simulink model "control_MI_dspic"  (R2018a)
settings: Solver=FixedStepAuto  StartTime=0.0  StopTime=4  FixedStep=Ts  RelTol=1e-5  EnableMultiTasking=on
PreLoadFcn:
  | inicio
InitFcn:
  | mex control_MI_dspic_main.c
values from neighbouring files (symbols this model uses):
  a = ((Llr+Lm).^2.*Rs + Lm.^2.*Rr) ./ (b.*(Llr+Lm))    [param_MI_LV.m]    (also in param_MI_VEU.m)
  A_s = 1.12    [param_veu.m]
  A_v = 1.4    [param_veu.m]
  B = 0.005752    [param_MI_LV.m]    (also in param_veu.m = 1.02)
  b = (Lls+Lm).*(Llr+Lm)-Lm.^2    [param_MI_LV.m]    (also in param_MI_VEU.m)
  B_s = (K_s/d_s)^(1/n_s)    (= 40.3936451136)    [param_veu.m]
  C = 0.68    [param_veu.m]
  C_d = 0.5    [param_veu.m]
  C_r = 0    [param_veu.m]
  C_s = 0.625    [param_veu.m]
  D_s = 1    [param_veu.m]
  eta_t = 0.9    [param_veu.m]
  g = 9.81    [param_veu.m]
  H = 0.47    [param_veu.m]
  H_a = H    (= 0.47)    [param_veu.m]
  J_m = 0.02    [param_veu.m]
  J_t = 0    [param_veu.m]
  J_wf = J_wr    (= 1.95)    [param_veu.m]
  J_wr = 1.95    [param_veu.m]
  L = 1.7    [param_veu.m]
  Lm = 0.00266    [param_MI_LV.m]    (also in param_MI_VEU.m = 0.003940447)
  Lr = (Llr + Lm)    (= 0.00277)    [param_MI_LV.m]    (also in param_MI_VEU.m = 0.004120686)
  Ls = (Lls + Lm)    (= 0.00277)    [param_MI_LV.m]    (also in param_MI_VEU.m = 0.004120686)
  m_v = 590    [param_veu.m]
  N_t = 10.3    [param_veu.m]
  P = 4    [param_MI_LV.m]    (also in param_MI_VEU.m)
  R = 0.268    [param_veu.m]
  ro_v = 1.225    [param_veu.m]
  Rr = 0.03471    [param_MI_LV.m]    (also in param_MI_VEU.m = 0.03841)
  Rs = 0.0697    [param_MI_LV.m]    (also in param_MI_VEU.m = 0.0274)
  sigma = (1- Lm^2/(Ls*Lr))    (= 0.0855669026076)    [param_MI_VEU.m]
  sigma_m = 0.005752    [param_veu.m]
  sigma_wf = sigma_wr    (= 0)    [param_veu.m]
  sigma_wr = 0    [param_veu.m]
  tita_w_0 = 0    [param_veu.m]
  Tr = (Llr+Lm)/Rr    (= 0.07980409104)    [param_MI_LV.m]    (also in param_MI_VEU.m = 0.107281593335)
  Ts = .5e-6    (= 5e-07)    [inicio.m]
  Tsc = 0.000054    (= 5.4e-05)    [inicio.m]    (also in param_MI_VEU.m)
  v_a_revancha = 0    [param_veu.m]
  v_x_0 = 00    (= 0)    [param_veu.m]
  w_w_0 = 0    [param_veu.m]
  x_x_0 = 0    [param_veu.m]
undefined symbols (not defined in the file or in its folder): DiscIntNeverNeededParam
libraries: powerlib x25, simulink x11, dspsigops x2, powerlib_meascontrol x1
(part 2 of 2)

== matlab function control_MI_dspic/mag1 ==
  data: VIndalpha output; VIndbeta output; Valpha input size=1; Vbeta input size=1; Ialpha input size=1; Ibeta input; dIalpha input; Esa output size=1; Esb output size=1; dIbeta input; mag output
% Facundo Aguilera

% Diseno de filtro para identificar fallas en sensores de corriente
% 2013


function [VIndalpha, VIndbeta, Esa, Esb, mag]    = fcn(Valpha, Vbeta, Ialpha, Ibeta, dIalpha, dIbeta)
    
    
    Rs = 0.0697;
    Lm = 0.00266;
    Lr = 0.00011+Lm;

    Sigma = 1 - Lm^2/Lr^2;
    
    Ls = Lr;

    
    VIndalpha = Sigma*Ls * dIalpha ;
    VIndbeta  = Sigma*Ls * dIbeta ;

    Esa		= 	Valpha -	Rs * Ialpha - VIndalpha;
    Esb		= 	Vbeta  -	Rs * Ibeta  - VIndbeta;

    mag = sqrt(Esa^2+Esb^2);

end

== matlab function control_MI_dspic/observador_bier/detector_a_adap_heun1 ==
  data: Valpha input size=1; Vbeta input size=1; i_q_ref input; i_d_ref input; omega_est input size=1; error output size=1; tita input
% Facundo Aguilera
% 2019


function error   = fcn(Valpha, Vbeta, i_q_ref, i_d_ref, omega_est, tita)

	Rs = 0.0697;
    Lm = 0.00266;
    Lr = 0.00011+Lm;
    sigma = 1 - Lm^2/Lr^2;
    Ls = Lr;

    Vd = Valpha * cos(tita) + Vbeta  * sin(tita);
    Vq = Vbeta  * cos(tita) - Valpha * sin(tita);
    
    error = (  Vd + omega_est*sigma*Ls*i_q_ref - Rs*i_d_ref );
    
    %ddelta = ( (omega_est<0)*2 +1)* ddelta;
 
 
 
end

== matlab function control_MI_dspic/VEU/Long/Embedded MATLAB Function ==
  data: v_x input; a_x_1 input; a_x output; w_wr input; w_wf input; F_xr output; L parameter; m_v parameter; C parameter; H parameter; H_a parameter; B parameter; A_s parameter; B_s parameter; C_s parameter; D_s parameter; C_d parameter; F_xf output; C_r parameter; ro_v parameter; A_v parameter; v_a_revancha parameter size=1; g parameter; fi_v input; R parameter; mu_r output; sigma_r output; F_roz output
function [a_x, F_xr,   F_xf, mu_r, sigma_r, F_roz] = veu(v_x ,a_x_1,w_wr, w_wf, L, m_v, C, H, H_a, B, A_s, B_s, C_s, D_s, C_d,  C_r, ro_v, A_v, v_a_revancha, g, fi_v, R)


% V aero
F_a = 1/2.*ro_v.*A_v.*C_d.*(v_x - v_a_revancha)^2;
F_r = m_v.*g.*C_r.*v_x;

% Fuerzas longitudinales
sigma_r = (R*w_wr - v_x) ./ max(abs([v_x R*w_wr 0.001]));

mu_pr = sign(sigma_r)*(A_s.*(1 - exp(-B_s.*abs(sigma_r))) + C_s.*sigma_r.^2 - D_s*abs(sigma_r) );


%%%% TEST 
% se usa a_x = a_w*R para probar sin pacejka
%a_xt = R*a_w;
%F_xrt = (a_xt*m_v + F_r + F_a + m_v*g*sin(fi_v))/2;
%%%% /TEST

% valores con Pacejka  
% F_Kr = m_v*g/L * (C*cos(fi_v) - H*sin(fi_v)) - H_a*F_a/L;
% a_xp = ((m_v.*(1+2.*mu_pr.*H./L)).^-1)  .*(  2.*mu_pr.*F_Kr - m_v.*g.*sin(fi_v) - F_a - F_r);




% Fuerzas normales
F_zf = 1/L .* ( m_v.*g.*(C*cos(fi_v) - H.*sin(fi_v)) - H_a.*F_a )- H*m_v.*a_x_1;
F_zr = 1/L .* ( m_v.*g.*(B.*cos(fi_v) + H.*sin(fi_v)) + H_a.*F_a  ) + H*m_v.*a_x_1;
F_xrp = mu_pr.*F_zr;

%%%% TEST 
%mu_tr = F_xrt/F_zr;
%%%% /TEST 


% selecciono las salidas Pacejka
mu_r = mu_pr;
a_x = ((m_v).^-1)  .*(  mu_pr.*F_zr - m_v.*g.*sin(fi_v) - F_a - F_r);
%a_x = a_xp;
F_xr = F_xrp;


% por el momento se desprecia el rozamiento de la rueda delantera
mu_f = 0;
F_xf = mu_f.*F_zf;
F_roz =  m_v.*g.*sin(fi_v) + F_a + F_r;


% Aceleracion
